simulink model "BR_FSM_Sim"  (R2026b)
settings: Solver=FixedStepDiscrete  StopTime=180  FixedStep=0.1
InitFcn:
  | load_br_signals
settings Model: Creator=adarsh4our  LastModifiedBy=adarsh4our

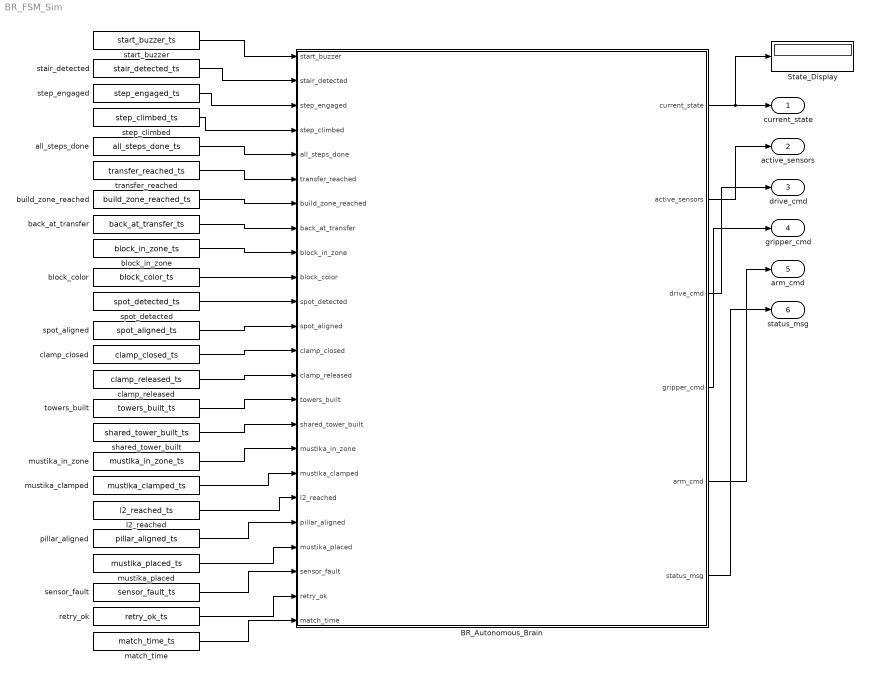
== system BR_FSM_Sim ==
  BR_Autonomous_Brain : Stateflow chart  TreatAsAtomicUnit=on
  State_Display : Display
  all_steps_done : FromWorkspace  VariableName=all_steps_done_ts  SampleTime=0.1  OutputAfterFinalValue=Holding final value
  back_at_transfer : FromWorkspace  VariableName=back_at_transfer_ts  SampleTime=0.1  OutputAfterFinalValue=Holding final value
  block_color : FromWorkspace  VariableName=block_color_ts  SampleTime=0.1  OutputAfterFinalValue=Holding final value
  block_in_zone : FromWorkspace  VariableName=block_in_zone_ts  SampleTime=0.1  OutputAfterFinalValue=Holding final value
  build_zone_reached : FromWorkspace  VariableName=build_zone_reached_ts  SampleTime=0.1  OutputAfterFinalValue=Holding final value
  clamp_closed : FromWorkspace  VariableName=clamp_closed_ts  SampleTime=0.1  OutputAfterFinalValue=Holding final value
  clamp_released : FromWorkspace  VariableName=clamp_released_ts  SampleTime=0.1  OutputAfterFinalValue=Holding final value
  l2_reached : FromWorkspace  VariableName=l2_reached_ts  SampleTime=0.1  OutputAfterFinalValue=Holding final value
  match_time : FromWorkspace  VariableName=match_time_ts  SampleTime=0.1  OutputAfterFinalValue=Holding final value
  mustika_clamped : FromWorkspace  VariableName=mustika_clamped_ts  SampleTime=0.1  OutputAfterFinalValue=Holding final value
  mustika_in_zone : FromWorkspace  VariableName=mustika_in_zone_ts  SampleTime=0.1  OutputAfterFinalValue=Holding final value
  mustika_placed : FromWorkspace  VariableName=mustika_placed_ts  SampleTime=0.1  OutputAfterFinalValue=Holding final value
  pillar_aligned : FromWorkspace  VariableName=pillar_aligned_ts  SampleTime=0.1  OutputAfterFinalValue=Holding final value
  retry_ok : FromWorkspace  VariableName=retry_ok_ts  SampleTime=0.1  OutputAfterFinalValue=Holding final value
  sensor_fault : FromWorkspace  VariableName=sensor_fault_ts  SampleTime=0.1  OutputAfterFinalValue=Holding final value
  shared_tower_built : FromWorkspace  VariableName=shared_tower_built_ts  SampleTime=0.1  OutputAfterFinalValue=Holding final value
  spot_aligned : FromWorkspace  VariableName=spot_aligned_ts  SampleTime=0.1  OutputAfterFinalValue=Holding final value
  spot_detected : FromWorkspace  VariableName=spot_detected_ts  SampleTime=0.1  OutputAfterFinalValue=Holding final value
  stair_detected : FromWorkspace  VariableName=stair_detected_ts  SampleTime=0.1  OutputAfterFinalValue=Holding final value
  start_buzzer : FromWorkspace  VariableName=start_buzzer_ts  SampleTime=0.1  OutputAfterFinalValue=Holding final value
  step_climbed : FromWorkspace  VariableName=step_climbed_ts  SampleTime=0.1  OutputAfterFinalValue=Holding final value
  step_engaged : FromWorkspace  VariableName=step_engaged_ts  SampleTime=0.1  OutputAfterFinalValue=Holding final value
  towers_built : FromWorkspace  VariableName=towers_built_ts  SampleTime=0.1  OutputAfterFinalValue=Holding final value
  transfer_reached : FromWorkspace  VariableName=transfer_reached_ts  SampleTime=0.1  OutputAfterFinalValue=Holding final value
  current_state : Outport
  active_sensors : Outport  Port=2
  drive_cmd : Outport  Port=3
  gripper_cmd : Outport  Port=4
  arm_cmd : Outport  Port=5
  status_msg : Outport  Port=6
  wires:
  start_buzzer/1 -> BR_Autonomous_Brain/1(start_buzzer)
  stair_detected/1 -> BR_Autonomous_Brain/2(stair_detected)
  step_engaged/1 -> BR_Autonomous_Brain/3(step_engaged)
  step_climbed/1 -> BR_Autonomous_Brain/4(step_climbed)
  all_steps_done/1 -> BR_Autonomous_Brain/5(all_steps_done)
  transfer_reached/1 -> BR_Autonomous_Brain/6(transfer_reached)
  build_zone_reached/1 -> BR_Autonomous_Brain/7(build_zone_reached)
  back_at_transfer/1 -> BR_Autonomous_Brain/8(back_at_transfer)
  block_in_zone/1 -> BR_Autonomous_Brain/9(block_in_zone)
  block_color/1 -> BR_Autonomous_Brain/10(block_color)
  spot_detected/1 -> BR_Autonomous_Brain/11(spot_detected)
  spot_aligned/1 -> BR_Autonomous_Brain/12(spot_aligned)
  clamp_closed/1 -> BR_Autonomous_Brain/13(clamp_closed)
  clamp_released/1 -> BR_Autonomous_Brain/14(clamp_released)
  towers_built/1 -> BR_Autonomous_Brain/15(towers_built)
  shared_tower_built/1 -> BR_Autonomous_Brain/16(shared_tower_built)
  mustika_in_zone/1 -> BR_Autonomous_Brain/17(mustika_in_zone)
  mustika_clamped/1 -> BR_Autonomous_Brain/18(mustika_clamped)
  l2_reached/1 -> BR_Autonomous_Brain/19(l2_reached)
  pillar_aligned/1 -> BR_Autonomous_Brain/20(pillar_aligned)
  mustika_placed/1 -> BR_Autonomous_Brain/21(mustika_placed)
  sensor_fault/1 -> BR_Autonomous_Brain/22(sensor_fault)
  retry_ok/1 -> BR_Autonomous_Brain/23(retry_ok)
  match_time/1 -> BR_Autonomous_Brain/24(match_time)
  BR_Autonomous_Brain/1(current_state) -> State_Display/1, current_state/1
  BR_Autonomous_Brain/2(active_sensors) -> active_sensors/1
  BR_Autonomous_Brain/3(drive_cmd) -> drive_cmd/1
  BR_Autonomous_Brain/4(gripper_cmd) -> gripper_cmd/1
  BR_Autonomous_Brain/5(arm_cmd) -> arm_cmd/1
  BR_Autonomous_Brain/6(status_msg) -> status_msg/1

== stateflow chart BR_FSM_Sim/BR_Autonomous_Brain ==
  settings: updateMethod=DISCRETE  sampleTime=0.1
  state ENGAGE_STEP_1
    entry:
    current_state=3;
    active_sensors=7;
    drive_cmd=1;
    gripper_cmd=0;
    arm_cmd=0;
    status_msg=2;
  state CLIMBING_L1
    entry:
    current_state=4;
    active_sensors=7;
    drive_cmd=1;
    gripper_cmd=0;
    arm_cmd=0;
    status_msg=3;
  state IDLE
    entry:
    current_state=1;
    active_sensors=0;
    drive_cmd=0;
    gripper_cmd=0;
    arm_cmd=0;
    status_msg=0;
  state NAV_TO_STAIR_1
    entry:
    current_state=2;
    active_sensors=7;
    drive_cmd=5;
    gripper_cmd=0;
    arm_cmd=0;
    status_msg=1;
  state PICK_BLOCK
    entry:
    current_state=8;
    active_sensors=20;
    drive_cmd=0;
    gripper_cmd=1;
    arm_cmd=3;
    status_msg=7;
  state WAIT_FOR_BLOCK
    entry:
    current_state=7;
    active_sensors=9;
    drive_cmd=0;
    gripper_cmd=0;
    arm_cmd=1;
    status_msg=6;
  state TRANSFER_READY
    entry:
    current_state=6;
    active_sensors=9;
    drive_cmd=5;
    gripper_cmd=0;
    arm_cmd=1;
    status_msg=5;
  state LEVEL_REACHED_L1
    entry:
    current_state=5;
    active_sensors=3;
    drive_cmd=0;
    gripper_cmd=0;
    arm_cmd=0;
    status_msg=4;
  state RECOVERY_RETRY
    entry:
    current_state=21;
    active_sensors=7;
    drive_cmd=4;
    gripper_cmd=2;
    arm_cmd=0;
    status_msg=-1;
  state RETURN_TO_TRANSFER
    entry:
    current_state=14;
    active_sensors=7;
    drive_cmd=4;
    gripper_cmd=0;
    arm_cmd=0;
    status_msg=13;
  state MATCH_COMPLETE
    entry:
    current_state=20;
    active_sensors=0;
    drive_cmd=0;
    gripper_cmd=0;
    arm_cmd=0;
    status_msg=99;
  state PLACE_BLOCK
    entry:
    current_state=12;
    active_sensors=24;
    drive_cmd=0;
    gripper_cmd=2;
    arm_cmd=2;
    status_msg=11;
  state DRIVE_TO_TOWER_AREA
    entry:
    current_state=9;
    active_sensors=7;
    drive_cmd=5;
    gripper_cmd=3;
    arm_cmd=4;
    status_msg=8;
  state DETECT_GREEN_SPOT
    entry:
    current_state=10;
    active_sensors=9;
    drive_cmd=2;
    gripper_cmd=3;
    arm_cmd=4;
    status_msg=9;
  state ALIGN_TO_SPOT
    entry:
    current_state=11;
    active_sensors=9;
    drive_cmd=3;
    gripper_cmd=3;
    arm_cmd=4;
    status_msg=10;
  state CHECK_SANCTUARY
    entry:
    current_state=13;
    active_sensors=0;
    drive_cmd=0;
    gripper_cmd=0;
    arm_cmd=0;
    status_msg=12;
  state PICK_MUSTIKA
    entry:
    current_state=16;
    active_sensors=24;
    drive_cmd=0;
    gripper_cmd=1;
    arm_cmd=3;
    status_msg=15;
  state WAIT_FOR_MUSTIKA
    entry:
    current_state=15;
    active_sensors=9;
    drive_cmd=0;
    gripper_cmd=0;
    arm_cmd=1;
    status_msg=14;
  state ENSHRINE_MUSTIKA
    entry:
    current_state=19;
    active_sensors=24;
    drive_cmd=0;
    gripper_cmd=2;
    arm_cmd=2;
    status_msg=18;
  state ALIGN_TO_PILLAR
    entry:
    current_state=18;
    active_sensors=9;
    drive_cmd=3;
    gripper_cmd=3;
    arm_cmd=4;
    status_msg=17;
  state NAV_TO_L2
    entry:
    current_state=17;
    active_sensors=7;
    drive_cmd=1;
    gripper_cmd=3;
    arm_cmd=0;
    status_msg=16;
  CLIMBING_L1 -> ENGAGE_STEP_1 [order 1] : [step_climbed == 1 && all_steps_done == 0]
  (default) -> IDLE
  IDLE -> NAV_TO_STAIR_1 : [start_buzzer == 1]
  NAV_TO_STAIR_1 -> ENGAGE_STEP_1 : [stair_detected == 1]
  ENGAGE_STEP_1 -> CLIMBING_L1 : [step_engaged == 1]
  CLIMBING_L1 -> LEVEL_REACHED_L1 [order 2] : [all_steps_done == 1]
  CLIMBING_L1 -> RECOVERY_RETRY [order 3] : [sensor_fault == 1]
  LEVEL_REACHED_L1 -> TRANSFER_READY : [transfer_reached == 1]
  TRANSFER_READY -> WAIT_FOR_BLOCK : [block_color > 0]
  PICK_BLOCK -> DRIVE_TO_TOWER_AREA [order 1] : [clamp_closed == 1]
  WAIT_FOR_BLOCK -> PICK_BLOCK [order 1] : [block_in_zone == 1 && block_color > 0]
  RETURN_TO_TRANSFER -> WAIT_FOR_BLOCK [order 2] : [back_at_transfer == 1]
  PICK_BLOCK -> RECOVERY_RETRY [order 2] : [sensor_fault == 1]
  WAIT_FOR_BLOCK -> MATCH_COMPLETE [order 2] : [match_time >= 180]
  ENSHRINE_MUSTIKA -> MATCH_COMPLETE : [mustika_placed == 1]
  RECOVERY_RETRY -> RETURN_TO_TRANSFER : [retry_ok == 1]
  DRIVE_TO_TOWER_AREA -> MATCH_COMPLETE [order 2] : [match_time >= 180]
  PLACE_BLOCK -> RECOVERY_RETRY [order 2] : [sensor_fault == 1]
  CHECK_SANCTUARY -> RETURN_TO_TRANSFER [order 1] : [towers_built < 2 || shared_tower_built == 0]
  RETURN_TO_TRANSFER -> MATCH_COMPLETE [order 1] : [match_time >= 180]
  NAV_TO_L2 -> RECOVERY_RETRY [order 2] : [sensor_fault == 1]
  ALIGN_TO_SPOT -> RECOVERY_RETRY [order 2] : [sensor_fault == 1]
  NAV_TO_L2 -> MATCH_COMPLETE [order 3] : [match_time >= 180]
  DRIVE_TO_TOWER_AREA -> DETECT_GREEN_SPOT [order 1] : [build_zone_reached == 1]
  DETECT_GREEN_SPOT -> ALIGN_TO_SPOT : [spot_detected == 1]
  ALIGN_TO_SPOT -> PLACE_BLOCK [order 1] : [spot_aligned == 1]
  PLACE_BLOCK -> CHECK_SANCTUARY [order 1] : [clamp_released == 1]
  CHECK_SANCTUARY -> WAIT_FOR_MUSTIKA [order 2] : [towers_built >= 2 && shared_tower_built == 1]
  ALIGN_TO_PILLAR -> ENSHRINE_MUSTIKA : [pillar_aligned == 1]
  PICK_MUSTIKA -> NAV_TO_L2 : [mustika_clamped == 1]
  WAIT_FOR_MUSTIKA -> PICK_MUSTIKA : [mustika_in_zone == 1]
  NAV_TO_L2 -> ALIGN_TO_PILLAR [order 1] : [l2_reached == 1]
  data: start_buzzer input double; stair_detected input double; step_engaged input double; step_climbed input double; all_steps_done input double; transfer_reached input double; build_zone_reached input double; back_at_transfer input double; block_in_zone input double; block_color input double; spot_detected input double; spot_aligned input double; clamp_closed input double; clamp_released input double; towers_built input double; shared_tower_built input double; mustika_in_zone input double; mustika_clamped input double; l2_reached input double; pillar_aligned input double; mustika_placed input double; sensor_fault input double; retry_ok input double; match_time input double; current_state output double; active_sensors output double; drive_cmd output double; gripper_cmd output double; arm_cmd output double; status_msg output double
  data start_buzzer settings: description=Match start signal (0/1)
  data stair_detected settings: description=LiDAR: stair edge detected within 20cm (0/1)
  data step_engaged settings: description=IMU: front wheel pitched up on riser (0/1)
  data step_climbed settings: description=IMU+Enc: pitch spike + encoder tick = 1 step done (0/1)
  data all_steps_done settings: description=Encoder: total step count reached target level (0/1)
  data transfer_reached settings: description=Encoder: arrived at Transfer Area position (0/1)
  data build_zone_reached settings: description=Encoder: arrived at target build zone (0/1)
  data back_at_transfer settings: description=Encoder: returned to Transfer Area (0/1)
  data block_in_zone settings: description=Depth Cam: block detected in Transfer Area (0/1)
  data block_color settings: description=Depth Cam: 1=Earth(Red/Blue) 2=Sky (for tower sequencing)
  data spot_detected settings: description=Depth Cam: green 500x500mm build spot found (0/1)
  data spot_aligned settings: description=Depth Cam: alignment error < 5mm (0/1)
  data clamp_closed settings: description=Limit switch: both jaws fully closed on block (0/1)
  data clamp_released settings: description=Limit switch: jaws fully open, block free (0/1)
  data towers_built settings: description=Counter: total complete towers (Earth+Earth+Sky)
  data shared_tower_built settings: description=Flag: 1 if tower placed in shared area (0/1)
  data mustika_in_zone settings: description=Depth Cam: Mustika (yellow/blue volleyball) detected (0/1)
  data mustika_clamped settings: description=Limit switch: jaws closed around volleyball (0/1)
  data l2_reached settings: description=Encoder+IMU: arrived at Level 2 (0/1)
  data pillar_aligned settings: description=Depth Cam: aligned over Central Pillar receptacle (0/1)
  data mustika_placed settings: description=Depth Cam: Mustika seated, no longer in gripper (0/1)
  data sensor_fault settings: description=Watchdog: any sensor timeout or OOB reading (0/1)
  data retry_ok settings: description=Encoder: BR returned to Retry Zone safely (0/1)
  data match_time settings: description=System clock: match elapsed time 0-180s
  data current_state settings: description=State ID 1-22
  data active_sensors settings: description=Sensor bitmask (see legend)
  data drive_cmd settings: description=0=STOP 1=CLIMB_STAIR 2=SCAN 3=FINE_POS 4=DESCEND 5=DRIVE_FWD
  data gripper_cmd settings: description=0=IDLE 1=CLOSE_CLAMP 2=OPEN_CLAMP 3=HOLD
  data arm_cmd settings: description=0=STOW 1=EXTEND 2=LOWER 3=LIFT 4=HOVER
  data status_msg settings: description=-1=FAULT 0=STANDBY 1-20=PROGRESS 99=VICTORY
